simulink model "SinV2relou"  (R2021a)
settings: Solver=VariableStepAuto  StartTime=0.0  StopTime=10.0  RelTol=1e-3
libraries: simulink x1
settings Model: Creator=lmeissne  LastModifiedBy=lmeissne

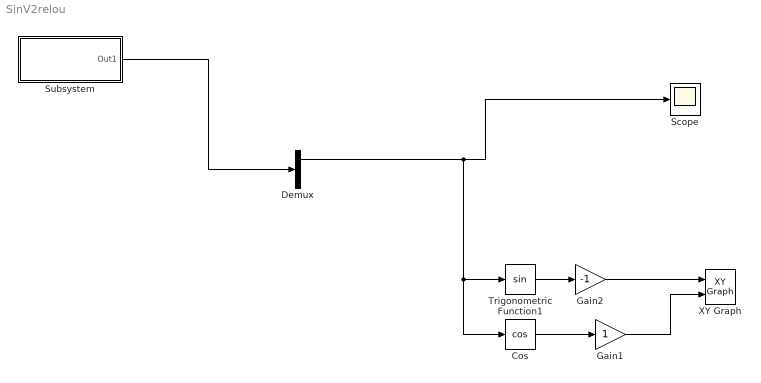
== system SinV2relou ==
  Cos : Trigonometry  Operator=cos
  Demux : Demux  Outputs=2
  Gain1 : Gain
  Gain2 : Gain  Gain=-1
  Scope : Scope
  Subsystem : Subsystem
  Trigonometric Function1 : Trigonometry
  XY Graph : simulink/Sinks/XY Graph  xmin=-1  xmax=1  ymin=-1  ymax=1  st=-1
  wires:
  Cos/1 -> Gain1/1
  Gain1/1 -> XY Graph/2
  Gain2/1 -> XY Graph/1
  Trigonometric Function1/1 -> Gain2/1
  Demux/1 -> Cos/1, Trigonometric Function1/1, Scope/1
  Subsystem/1(Out1) -> Demux/1

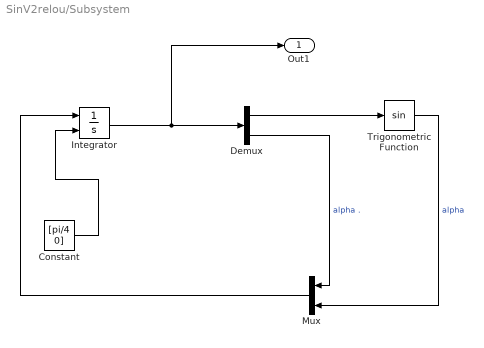
== system SinV2relou/Subsystem ==
  Constant : Constant  Value=[pi/4 0]  VectorParams1D=off
  Demux : Demux  Outputs=2
  Integrator : Integrator  InitialConditionSource=external
  Mux : Mux  Inputs=2
  Trigonometric Function : Trigonometry
  Out1 : Outport
  wires:
  Constant/1 -> Integrator/2
  Integrator/1 -> Out1/1, Demux/1
  Demux/1 -> Trigonometric Function/1
  Trigonometric Function/1 -> Mux/2  "alpha"
  Demux/2 -> Mux/1  "alpha ."
  Mux/1 -> Integrator/1
